simulink model "SplineGenerator"  (R2016b)
settings: Solver=VariableStepAuto  StartTime=0.0  StopTime=10.0  RelTol=1e-3
libraries: GaitGenerationLibrary x1
settings Model: Creator=march  LastModifiedBy=march

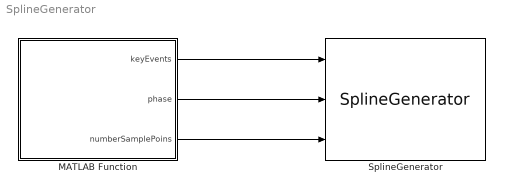
== system SplineGenerator ==
  MATLAB Function : MATLAB Function  TreatAsAtomicUnit=on
  SplineGenerator : GaitGenerationLibrary/SplineGenerator
  wires:
  MATLAB Function/1(keyEvents) -> SplineGenerator/1
  MATLAB Function/2(phase) -> SplineGenerator/2
  MATLAB Function/3(numberSamplePoins) -> SplineGenerator/3

== matlab function SplineGenerator/MATLAB Function ==
  data: keyEvents output; phase output; numberSamplePoins output
function [keyEvents, phase, numberSamplePoins] = fcn()

keyEvents = [0, 0, 0; ...
20, 40, -1; ...
40, 30,-1; ...
60,-10,0; ...
80,-10,1; ...
100,0,0];

phase = [0:0.1:100]';

numberSamplePoins = 100;
end
